simulink model "GenOptRockerMomtryDisHndlr_TestSupport"  (R2017b)
settings: configuration reference "JD_ConfigsetAUTOSARMulti10msec" (kept outside this file)
undefined symbols (not defined in the file): P_Std_ReturnType
settings Model: Creator=KIH3CPW  LastModifiedBy=KIH3CPW
settings ConfigSetRef: SourceLocation=Base Workspace

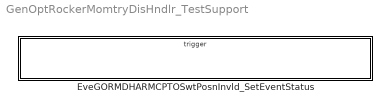
== system GenOptRockerMomtryDisHndlr_TestSupport ==
  EveGORMDHARMCPTOSwtPosnInvld_SetEventStatus : Subsystem  TreatAsAtomicUnit=on

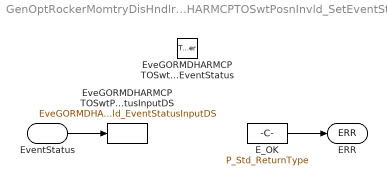
== system GenOptRockerMomtryDisHndlr_TestSupport/EveGORMDHARMCPTOSwtPosnInvld_SetEventStatus ==
  EveGORMDHARMCPTOSwtPosnInvld_SetEventStatus : TriggerPort  TriggerType=function-call  IsSimulinkFunction=on  FunctionName=EveGORMDHARMCPTOSwtPosnInvld_SetEventStatus  VariantControl=(inherit)
  E_OK : Constant  Value=P_Std_ReturnType
  EveGORMDHARMCPTOSwtPosnInvld_EventStatusInputDS : DataStoreWrite  DataStoreName=EveGORMDHARMCPTOSwtPosnInvld_EventStatusInputDS
  EventStatus : ArgIn  DisableCoverage=on  OutDataTypeStr=Enum: Dem_EventStatusType  ArgumentName=EventStatus
  ERR : ArgOut  DisableCoverage=on  OutDataTypeStr=Std_ReturnType  ArgumentName=ERR
  wires:
  EventStatus/1 -> EveGORMDHARMCPTOSwtPosnInvld_EventStatusInputDS/1
  E_OK/1 -> ERR/1
